simulink subsystem "Robot_Control_sub"  (R2023b)
settings: Solver=VariableStepAuto  StartTime=0.0  StopTime=10.0  RelTol=1e-3
libraries: Autonomous_lib x1, Disabled_lib x1, Teleop_lib x1, Test_lib x1
settings Model: Creator=USER  LastModifiedBy=ander

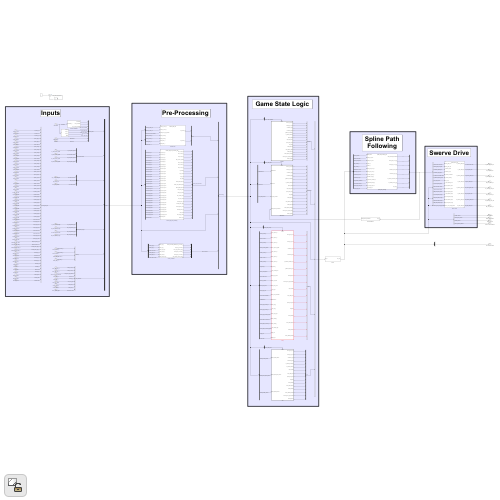
[thumbnail: Simulink's stored preview of the top-level diagram]
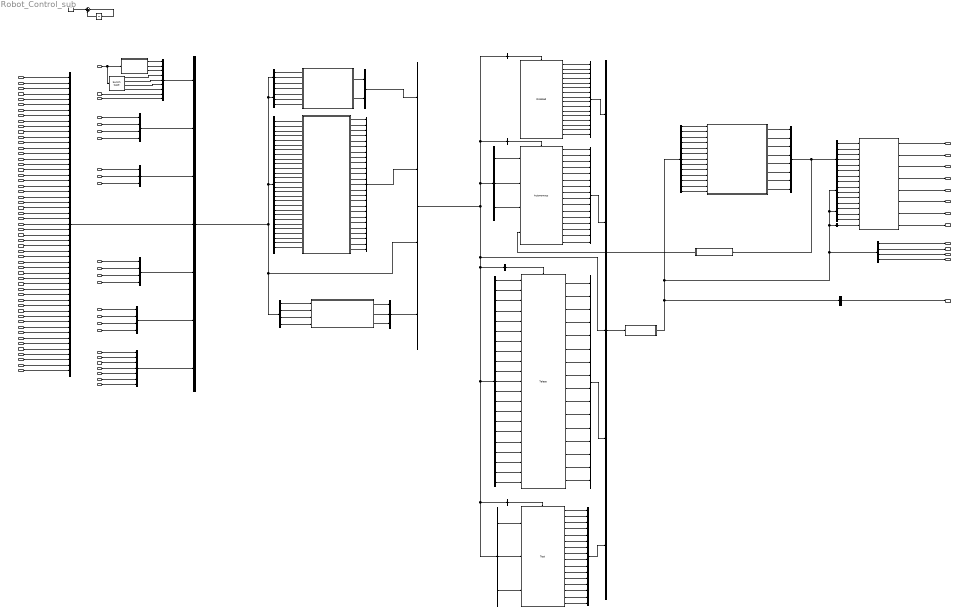
== system Robot_Control_sub ==
  note: Game State Logic
  note: Swerve Drive
  note: Inputs
  note: Pre-Processing
  note: Spline Path
      | Following
  GameState : Inport
  IsBlueAlliance : Inport  Port=2
  MatchTime : Inport  Port=3
  Joystick_Left_X : Inport  Port=4
  Joystick_Left_Y : Inport  Port=5
  Joystick_Left_Z : Inport  Port=6
  Joystick_Right_X : Inport  Port=7
  Joystick_Right_Y : Inport  Port=8
  Joystick_Right_Z : Inport  Port=9
  Joystick_Left_B1 : Inport  Port=10
  Joystick_Left_B2 : Inport  Port=11
  Joystick_Left_B3 : Inport  Port=12
  Joystick_Left_B4 : Inport  Port=13
  Joystick_Left_B5 : Inport  Port=14
  Joystick_Left_B6 : Inport  Port=15
  Joystick_Left_B7 : Inport  Port=16
  Joystick_Left_B8 : Inport  Port=17
  Joystick_Left_B9 : Inport  Port=18
  Joystick_Left_B10 : Inport  Port=19
  Joystick_Left_B11 : Inport  Port=20
  Joystick_Left_B12 : Inport  Port=21
  Joystick_Left_B13 : Inport  Port=22
  Joystick_Left_B14 : Inport  Port=23
  Joystick_Left_B15 : Inport  Port=24
  Joystick_Left_B16 : Inport  Port=25
  Joystick_Left_POV : Inport  Port=26
  Joystick_Right_B1 : Inport  Port=27
  Joystick_Right_B2 : Inport  Port=28
  Joystick_Right_B3 : Inport  Port=29
  Joystick_Right_B4 : Inport  Port=30
  Joystick_Right_B5 : Inport  Port=31
  Joystick_Right_B6 : Inport  Port=32
  Joystick_Right_B7 : Inport  Port=33
  Joystick_Right_B8 : Inport  Port=34
  Joystick_Right_B9 : Inport  Port=35
  Joystick_Right_B10 : Inport  Port=36
  Joystick_Right_B11 : Inport  Port=37
  Joystick_Right_B12 : Inport  Port=38
  Joystick_Right_B13 : Inport  Port=39
  Joystick_Right_B14 : Inport  Port=40
  Joystick_Right_B15 : Inport  Port=41
  Joystick_Right_B16 : Inport  Port=42
  Joystick_Right_POV : Inport  Port=43
  Gamepad_Stick_Left_X : Inport  Port=44
  Gamepad_Stick_Left_Y : Inport  Port=45
  Gamepad_Stick_Right_X : Inport  Port=46
  Gamepad_Stick_Right_Y : Inport  Port=47
  Gamepad_B1_A : Inport  Port=48
  Gamepad_B2_B : Inport  Port=49
  Gamepad_B3_X : Inport  Port=50
  Gamepad_B4_Y : Inport  Port=51
  Gamepad_LB : Inport  Port=52
  Gamepad_LT : Inport  Port=53
  Gamepad_RB : Inport  Port=54
  Gamepad_RT : Inport  Port=55
  Gamepad_Back : Inport  Port=56
  Gamepad_Start : Inport  Port=57
  Gamepad_POV : Inport  Port=58
  FL_Drive_Motor_Speed : Inport  Port=59
  FR_Drive_Motor_Speed : Inport  Port=60
  BL_Drive_Motor_Speed : Inport  Port=61
  BR_Drive_Motor_Speed : Inport  Port=62
  Gyro_Angle_Field_rad : Inport  Port=63
  Gyro_Angle_rad : Inport  Port=64
  Auto_Start_Position : Inport  Port=65
  FL_Steer_Module_Angle : Inport  Port=66
  FR_Steer_Module_Angle : Inport  Port=67
  BL_Steer_Module_Angle : Inport  Port=68
  BR_Steer_Module_Angle : Inport  Port=69
  Odom_Position_X : Inport  Port=70
  Odom_Position_Y : Inport  Port=71
  Odom_Delta_X : Inport  Port=72
  Odom_Delta_Y : Inport  Port=73
  Vision_Current_Pipeline : Inport  Port=74
  Vision_RobotPoseFieldSpace_X : Inport  Port=75
  Vision_RobotPoseFieldSpace_Y : Inport  Port=76
  Vision_Num_Tags_Detected : Inport  Port=77
  Vision_c1TargetPoseRobotSpace_X : Inport  Port=78
  Vision_c1TargetPoseRobotSpace_Y : Inport  Port=79
  Vision_c1TargetPoseRobotSpace_A : Inport  Port=80
  Autonomous : Autonomous_lib/Autonomous  SystemSampleTime=-1  VariantActivationTime=update diagram  AllowFlexibleInterface=on  Latency=0  AutoFrameSizeCalculation=off
  Bus Creator : BusCreator  Inputs=9
  Bus Creator{1..2,4,12} (4 alike) : BusCreator  Inputs=16
  Bus Creator11 : BusCreator  Inputs=7
  Bus Creator13 : BusCreator  Inputs=8
  Bus Creator14 : BusCreator  Inputs=3
  Bus Creator{7..9,17} (4 alike) : BusCreator  Inputs=4
  Bus Creator18 : BusCreator  Inputs=7
  Bus Creator19 : BusCreator  Inputs=2
  Bus Creator21 : BusCreator  Inputs=3
  Bus Creator24 : BusCreator  Inputs=25
  Bus Creator3 : BusCreator  Inputs=5
  Bus Creator5 : BusCreator  Inputs=55
  Bus Selector : BusSelector  OutputSignals=Steering_Abs_Cmd_SPF,Steering_Rel_Cmd_SPF,Translation_Speed_SPF,Translation_Angle_SPF,Is_Absolute_Translation_SPF,Is_Absolute_Steering_SPF,Gyro_Angle_SPF
  Bus Selector1 : BusSelector  OutputSignals=Odometry.Odom_Position_X,Odometry.Odom_Position_Y,Odometry.Odom_Delta_X,Odometry.Odom_Delta_Y
  Bus Selector13 : BusSelector  OutputSignals=Human_Inputs_Raw.Joystick_Left_X,Human_Inputs_Raw.Joystick_Left_Y,Human_Inputs_Raw.Joystick_Left_Z,Human_Inputs_Raw.Joystick_Right_X,Human_Inputs_Raw.Joystick_Right_Y,Human_Inputs_Raw.Joystick_Right_Z,Human_Inputs_Raw.Joystick_Left_B1,Human_Inputs_Raw.Joystick_Left_B2,Human_Inputs_Raw.Joystick_Left_B3,Human_Inputs_Raw.Joystick_Left_B4,Human_Inputs_Raw.Joystick_Left_B5,Human_Inputs_Raw.Joystick_Left_B7,Human_Inputs_Raw.Joystick_Left_B8,Human_Inputs_Raw.Joystick_Left_B11,Human_Inputs_Raw.Joystick_Left_B12,Human_Inputs_Raw.Joystick_Left_B13,Human_Inputs_Raw.Joystick_Left_POV,Human_Inputs_Raw.Joystick_Right_B2,Human_Inputs_Raw.Joystick_Right_B3,Human_Inputs_Raw.Joystick_Right_B4,Human_Inputs_Raw.Joystick_Right_B5,Human_Inputs_Raw.Joystick_Right_B6,Human_Inputs_Raw.Joystick_Right_B7,Human_Inputs_Raw.Joystick_Right_B8,Human_Inputs_Raw.Joystick_Right_B9,Human_Inputs_Raw.Joystick_Right_B10,Human_Inputs_Raw.Joystick_Right_POV,Human_Inputs_Raw.Gamepad_POV
  Bus Selector16 : BusSelector  OutputSignals=Human_Inputs_Processed.Button_Enable_Wheels,Human_Inputs_Processed.Button_Reset_Wheel_Offsets,Human_Inputs_Processed.Button_Disable_Wheels
  Bus Selector18 : BusSelector  OutputSignals=Enable_Wheels,Reset_Wheel_Offsets,Disable_Wheels,Swerve_Motors_Disabled
  Bus Selector2 : BusSelector  OutputSignals=Inputs.Game_States.Game_State_Teleop
  Bus Selector20 : BusSelector  OutputSignals=Vision_Estimates.Vision_Current_Pipeline,Vision_Estimates.Vision_c1TargetPoseRobotSpace_X,Vision_Estimates.Vision_c1TargetPoseRobotSpace_Y,Vision_Estimates.Vision_c1TargetPoseRobotSpace_A
  Bus Selector21 : BusSelector  OutputSignals=Swerve_Drive_Integral_Enable
  Bus Selector23 : BusSelector  OutputSignals=Desired_Pipeline  OutputAsBus=on
  Bus Selector3 : BusSelector  OutputSignals=Vision_Estimates.Vision_RobotPoseFieldSpace_X,Vision_Estimates.Vision_RobotPoseFieldSpace_Y,Vision_Estimates.Vision_Num_Tags_Detected
  Bus Selector4 : BusSelector  OutputSignals=Inputs.Game_States.Game_State_Auto
  Bus Selector41 : BusSelector  OutputSignals=Human_Inputs_Processed.Drive_Joystick_X,Human_Inputs_Processed.Drive_Joystick_Y,Human_Inputs_Processed.Drive_Joystick_Z,Human_Inputs_Processed.Drive_Joystick_Z_Mode,Human_Inputs_Processed.Steer_Joystick_X,Human_Inputs_Processed.Steer_Joystick_Y,Human_Inputs_Processed.Steer_Joystick_Z,Human_Inputs_Processed.Is_Boosting,Human_Inputs_Processed.Face_Toward_Driver,Human_Inputs_Processed.Face_Right_Driver,Human_Inputs_Processed.Face_Left_Driver,Human_Inputs_Processed.Face_Away_Driver,Inputs.Gyro.Gyro_Angle_rad,Inputs.Game_States.Prev_Active_GameState,Inputs.Game_States.IsBlueAlliance,Inputs.Vision_Estimates.Vision_Current_Pipeline,Vision_Corrected.Vision_c1TPRS_Corrected_X,Vision_Corrected.Vision_c1TPRS_Corrected_Y,Vision_Corrected.Vision_c1TPRS_Corrected_A,Human_Inputs_Processed.Align_Left,Human_Inputs_Processed.Align_Right
  Bus Selector50 : BusSelector  OutputSignals=PreProcessing.Inputs.Drive_Motor_Speeds.FL_Drive_Motor_Speed,PreProcessing.Inputs.Drive_Motor_Speeds.FR_Drive_Motor_Speed,PreProcessing.Inputs.Drive_Motor_Speeds.BL_Drive_Motor_Speed,PreProcessing.Inputs.Drive_Motor_Speeds.BR_Drive_Motor_Speed
  Bus Selector52 : BusSelector  OutputSignals=PreProcessing.Inputs.Steer_Module_Angles.FL_Steer_Module_Angle,PreProcessing.Inputs.Steer_Module_Angles.FR_Steer_Module_Angle,PreProcessing.Inputs.Steer_Module_Angles.BL_Steer_Module_Angle,PreProcessing.Inputs.Steer_Module_Angles.BR_Steer_Module_Angle
  Bus Selector59 : BusSelector  OutputSignals=Inputs.Game_States.IsBlueAlliance,Inputs.Game_States.MatchTime,Inputs.Gyro.Auto_Start_Position
  Bus Selector6 : BusSelector  OutputSignals=Inputs.Game_States.Game_State_Disabled
  Bus Selector8 : BusSelector  OutputSignals=Inputs.Game_States.Game_State_Test
  Bus Selector9 : BusSelector  OutputSignals=Spline_Enable,Spline_Ref_Poses,Spline_Num_Poses,PreProcessing.EKF.KF_Position_X,PreProcessing.EKF.KF_Position_Y,Steering_Abs_Cmd,Steering_Rel_Cmd,Translation_Speed,Translation_Angle,Is_Absolute_Translation,Is_Absolute_Steering,PreProcessing.Inputs.Gyro.Gyro_Angle_Field_rad,PreProcessing.Inputs.Gyro.Gyro_Angle_rad
  Constant2 : Constant
  Disabled : Disabled_lib/Disabled  SystemSampleTime=-1  VariantActivationTime=update diagram  AllowFlexibleInterface=on  Latency=0  AutoFrameSizeCalculation=off
  Human_Input_Pre_Processing : Subsystem  ReferencedSubsystem=Human_Input_Pre_Processing_sub
  Internal Feedback : Subsystem
  Kalman_Filter : Subsystem  ReferencedSubsystem=Kalman_Filter_sub
  Merge : Subsystem
  Previous GameState : Subsystem
  Spline_Path_Following : Subsystem  ReferencedSubsystem=Spline_Path_Following_sub
  Sum : Sum  Inputs=|++
  Swerve_Drive : Subsystem  ReferencedSubsystem=Swerve_Drive_sub
  Switch Case : SwitchCase  CaseConditions={0,1,2}
  Teleop : Teleop_lib/Teleop  SystemSampleTime=-1  VariantActivationTime=update diagram  AllowFlexibleInterface=on  Latency=0  AutoFrameSizeCalculation=off
  Test : Test_lib/Test  SystemSampleTime=-1  VariantActivationTime=update diagram  AllowFlexibleInterface=on  Latency=0  AutoFrameSizeCalculation=off
  Unit Delay1 : UnitDelay  SampleTime=-1  HasFrameUpgradeWarning=on
  Vision_Corrections : Subsystem  ReferencedSubsystem=Vision_Corrections_sub
  FL_Steering_Motor_DC : Outport
  FL_Drive_Motor_DC : Outport  Port=2
  FR_Steering_Motor_DC : Outport  Port=3
  FR_Drive_Motor_DC : Outport  Port=4
  BL_Steering_Motor_DC : Outport  Port=5
  BL_Drive_Motor_DC : Outport  Port=6
  BR_Steering_Motor_DC : Outport  Port=7
  BR_Drive_Motor_DC : Outport  Port=8
  Enable_Wheels : Outport  Port=9
  Reset_Wheel_Offsets : Outport  Port=10
  Disable_Wheels : Outport  Port=11
  Swerve_Motors_Disabled : Outport  Port=12
  Vision_Desired_Pipeline : Outport  Port=13
  wires:
  Bus Creator4/1 -> Bus Creator3/1  "Disabled"
  Bus Creator1/1 -> Bus Creator3/2  "Autonomous"
  Bus Creator2/1 -> Bus Creator3/4  "Teleop"
  Switch Case/1 -> Bus Creator/4  "Game_State_Disabled"
  Switch Case/2 -> Bus Creator/5  "Game_State_Auto"
  Switch Case/3 -> Bus Creator/6  "Game_State_Teleop"
  GameState/1 -> Previous GameState/1(GameState_in), Switch Case/1  "GameState"
  Bus Creator12/1 -> Bus Creator3/5  "Test"
  Switch Case/4 -> Bus Creator/7  "Game_State_Test"
  FL_Drive_Motor_Speed/1 -> Bus Creator7/1  "FL_Drive_Motor_Speed"
  FR_Drive_Motor_Speed/1 -> Bus Creator7/2  "FR_Drive_Motor_Speed"
  BL_Drive_Motor_Speed/1 -> Bus Creator7/3  "BL_Drive_Motor_Speed"
  BR_Drive_Motor_Speed/1 -> Bus Creator7/4  "BR_Drive_Motor_Speed"
  Bus Creator/1 -> Bus Creator11/1  "Game_States"
  Bus Selector2/1 -> Teleop/Action  "<Game_State_Teleop>"
  Bus Selector4/1 -> Autonomous/Action  "<Game_State_Auto>"
  Bus Selector6/1 -> Disabled/Action  "<Game_State_Disabled>"
  Bus Selector8/1 -> Test/Action  "<Game_State_Test>"
  Bus Selector50/4 -> Swerve_Drive/11  "<BR_Drive_Motor_Speed>"
  Bus Selector50/3 -> Swerve_Drive/10  "<BL_Drive_Motor_Speed>"
  Bus Selector50/2 -> Swerve_Drive/9  "<FR_Drive_Motor_Speed>"
  Bus Selector50/1 -> Swerve_Drive/8  "<FL_Drive_Motor_Speed>"
  Swerve_Drive/1 -> FL_Steering_Motor_DC/1
  Swerve_Drive/2 -> FL_Drive_Motor_DC/1
  Swerve_Drive/3 -> FR_Steering_Motor_DC/1
  Swerve_Drive/4 -> FR_Drive_Motor_DC/1
  Swerve_Drive/5 -> BL_Steering_Motor_DC/1
  Swerve_Drive/6 -> BL_Drive_Motor_DC/1
  Swerve_Drive/7 -> BR_Steering_Motor_DC/1
  Swerve_Drive/8 -> BR_Drive_Motor_DC/1
  Joystick_Left_B1/1 -> Bus Creator5/7  "Joystick_Left_B1"
  Gyro_Angle_Field_rad/1 -> Bus Creator14/1  "Gyro_Angle_Field_rad"
  Gyro_Angle_rad/1 -> Bus Creator14/2  "Gyro_Angle_rad"
  Bus Creator11/1 -> Bus Creator17/3, Bus Selector20/1, Bus Selector1/1, Bus Selector3/1, Bus Selector13/1  "Inputs"
  Bus Selector52/1 -> Swerve_Drive/12  "<FL_Steer_Module_Angle>"
  Bus Selector52/2 -> Swerve_Drive/13  "<FR_Steer_Module_Angle>"
  Bus Selector52/3 -> Swerve_Drive/14  "<BL_Steer_Module_Angle>"
  Bus Selector52/4 -> Swerve_Drive/15  "<BR_Steer_Module_Angle>"
  Merge/1(Bus_Out) -> Bus Selector23/1, Bus Selector9/1, Bus Selector18/1, Bus Selector21/1, Bus Selector52/1, Bus Selector50/1
  Bus Creator3/1 -> Merge/1(Bus_In)
  Bus Selector9/1 -> Spline_Path_Following/1  "<Spline_Enable>"
  Bus Selector9/2 -> Spline_Path_Following/2  "<Spline_Ref_Poses>"
  Bus Selector9/3 -> Spline_Path_Following/3  "<Spline_Num_Poses>"
  Bus Selector9/6 -> Spline_Path_Following/6  "<Steering_Abs_Cmd>"
  Bus Selector9/7 -> Spline_Path_Following/7  "<Steering_Rel_Cmd>"
  Bus Selector9/8 -> Spline_Path_Following/8  "<Translation_Speed>"
  Bus Selector9/9 -> Spline_Path_Following/9  "<Translation_Angle>"
  Bus Selector9/10 -> Spline_Path_Following/10  "<Is_Absolute_Translation>"
  Bus Selector9/11 -> Spline_Path_Following/11  "<Is_Absolute_Steering>"
  Spline_Path_Following/2 -> Bus Creator13/2
  Spline_Path_Following/3 -> Bus Creator13/3
  Spline_Path_Following/4 -> Bus Creator13/4
  Spline_Path_Following/5 -> Bus Creator13/5
  Spline_Path_Following/6 -> Bus Creator13/6
  Spline_Path_Following/7 -> Bus Creator13/7
  Bus Creator13/1 -> Bus Selector/1, Internal Feedback/1(Bus_In)
  Bus Selector/5 -> Swerve_Drive/5  "<Is_Absolute_Translation_SPF>"
  Bus Selector/4 -> Swerve_Drive/4  "<Translation_Angle_SPF>"
  Bus Selector/6 -> Swerve_Drive/6  "<Is_Absolute_Steering_SPF>"
  Bus Selector/3 -> Swerve_Drive/3  "<Translation_Speed_SPF>"
  Bus Selector/2 -> Swerve_Drive/2  "<Steering_Rel_Cmd_SPF>"
  Bus Selector/1 -> Swerve_Drive/1  "<Steering_Abs_Cmd_SPF>"
  Spline_Path_Following/1 -> Bus Creator13/1
  Vision_RobotPoseFieldSpace_X/1 -> Bus Creator18/2  "Vision_RobotPoseFieldSpace_X"
  Vision_RobotPoseFieldSpace_Y/1 -> Bus Creator18/3  "Vision_RobotPoseFieldSpace_Y"
  Vision_Num_Tags_Detected/1 -> Bus Creator18/4  "Vision_Num_Tags_Detected"
  Bus Selector1/3 -> Kalman_Filter/6  "<Odom_Delta_X>"
  Bus Selector1/4 -> Kalman_Filter/7  "<Odom_Delta_Y>"
  Bus Selector3/3 -> Kalman_Filter/3  "<Vision_Num_Tags_Detected>"
  Bus Selector3/2 -> Kalman_Filter/2  "<Vision_RobotPoseFieldSpace_Y>"
  Bus Selector3/1 -> Kalman_Filter/1  "<Vision_RobotPoseFieldSpace_X>"
  Kalman_Filter/1 -> Bus Creator19/1
  Kalman_Filter/2 -> Bus Creator19/2
  Bus Selector9/4 -> Spline_Path_Following/4  "<KF_Position_X>"
  Bus Selector9/5 -> Spline_Path_Following/5  "<KF_Position_Y>"
  Bus Creator19/1 -> Bus Creator17/1  "EKF"
  Bus Selector1/2 -> Kalman_Filter/5  "<Odom_Position_Y>"
  Bus Selector1/1 -> Kalman_Filter/4  "<Odom_Position_X>"
  Joystick_Left_B4/1 -> Bus Creator5/10  "Joystick_Left_B4"
  Joystick_Left_B3/1 -> Bus Creator5/9  "Joystick_Left_B3"
  Joystick_Left_B2/1 -> Bus Creator5/8  "Joystick_Left_B2"
  Bus Selector13/4 -> Human_Input_Pre_Processing/4  "<Joystick_Right_X>"
  Bus Selector13/5 -> Human_Input_Pre_Processing/5  "<Joystick_Right_Y>"
  Bus Selector13/1 -> Human_Input_Pre_Processing/1  "<Joystick_Left_X>"
  Bus Selector13/3 -> Human_Input_Pre_Processing/3  "<Joystick_Left_Z>"
  Bus Selector13/2 -> Human_Input_Pre_Processing/2  "<Joystick_Left_Y>"
  Bus Selector13/6 -> Human_Input_Pre_Processing/6  "<Joystick_Right_Z>"
  Bus Selector13/7 -> Human_Input_Pre_Processing/7  "<Joystick_Left_B1>"
  Bus Selector13/8 -> Human_Input_Pre_Processing/8  "<Joystick_Left_B2>"
  Bus Selector13/9 -> Human_Input_Pre_Processing/9  "<Joystick_Left_B3>"
  Bus Selector13/10 -> Human_Input_Pre_Processing/10  "<Joystick_Left_B4>"
  Joystick_Left_Y/1 -> Bus Creator5/2  "Joystick_Left_Y"
  Joystick_Left_X/1 -> Bus Creator5/1  "Joystick_Left_X"
  Joystick_Left_Z/1 -> Bus Creator5/3  "Joystick_Left_Z"
  Joystick_Right_X/1 -> Bus Creator5/4  "Joystick_Right_X"
  Joystick_Right_Y/1 -> Bus Creator5/5  "Joystick_Right_Y"
  Joystick_Right_Z/1 -> Bus Creator5/6  "Joystick_Right_Z"
  Bus Creator24/1 -> Bus Creator17/2  "Human_Inputs_Processed"
  Bus Creator17/1 -> Bus Selector59/1, Bus Selector4/1, Bus Selector6/1, Bus Creator3/3, Bus Selector2/1, Bus Selector41/1, Bus Selector8/1, Bus Selector16/1  "PreProcessing"
  Bus Creator18/1 -> Bus Creator11/7  "Vision_Estimates"
  Internal Feedback/1(Robot_Reached_Destination) -> Autonomous/4
  Vision_c1TargetPoseRobotSpace_X/1 -> Bus Creator18/5  "Vision_c1TargetPoseRobotSpace_X"
  Vision_c1TargetPoseRobotSpace_Y/1 -> Bus Creator18/6  "Vision_c1TargetPoseRobotSpace_Y"
  Previous GameState/1(GameState) -> Bus Creator/1
  Previous GameState/3(Prev_Active_GameState) -> Bus Creator/3
  IsBlueAlliance/1 -> Bus Creator/8  "IsBlueAlliance"
  Bus Selector9/12 -> Spline_Path_Following/12  "<Gyro_Angle_Field_rad>"
  Bus Selector9/13 -> Spline_Path_Following/13  "<Gyro_Angle_rad>"
  Spline_Path_Following/8 -> Bus Creator13/8
  Bus Selector/7 -> Swerve_Drive/7  "<Gyro_Angle_SPF>"
  Bus Selector59/1 -> Autonomous/1  "<IsBlueAlliance>"
  Bus Selector18/2 -> Reset_Wheel_Offsets/1  "<Reset_Wheel_Offsets>"
  Bus Selector18/3 -> Disable_Wheels/1  "<Disable_Wheels>"
  Bus Selector18/4 -> Swerve_Motors_Disabled/1  "<Swerve_Motors_Disabled>"
  Bus Selector18/1 -> Enable_Wheels/1  "<Enable_Wheels>"
  Bus Selector16/1 -> Test/1  "<Button_Enable_Wheels>"
  Bus Selector16/2 -> Test/2  "<Button_Reset_Wheel_Offsets>"
  Bus Selector16/3 -> Test/3  "<Button_Disable_Wheels>"
  Joystick_Left_B5/1 -> Bus Creator5/11  "Joystick_Left_B5"
  Joystick_Left_B6/1 -> Bus Creator5/12  "Joystick_Left_B6"
  Joystick_Left_B7/1 -> Bus Creator5/13  "Joystick_Left_B7"
  Joystick_Left_B8/1 -> Bus Creator5/14  "Joystick_Left_B8"
  Joystick_Left_B9/1 -> Bus Creator5/15  "Joystick_Left_B9"
  Joystick_Left_B10/1 -> Bus Creator5/16  "Joystick_Left_B10"
  Joystick_Left_B11/1 -> Bus Creator5/17  "Joystick_Left_B11"
  Joystick_Left_B12/1 -> Bus Creator5/18  "Joystick_Left_B12"
  Joystick_Left_B13/1 -> Bus Creator5/19  "Joystick_Left_B13"
  Joystick_Left_B14/1 -> Bus Creator5/20  "Joystick_Left_B14"
  Joystick_Left_B15/1 -> Bus Creator5/21  "Joystick_Left_B15"
  Joystick_Left_B16/1 -> Bus Creator5/22  "Joystick_Left_B16"
  Joystick_Left_POV/1 -> Bus Creator5/23  "Joystick_Left_POV"
  Joystick_Right_B1/1 -> Bus Creator5/24  "Joystick_Right_B1"
  Joystick_Right_B2/1 -> Bus Creator5/25  "Joystick_Right_B2"
  Joystick_Right_B3/1 -> Bus Creator5/26  "Joystick_Right_B3"
  Joystick_Right_B4/1 -> Bus Creator5/27  "Joystick_Right_B4"
  Joystick_Right_B5/1 -> Bus Creator5/28  "Joystick_Right_B5"
  Joystick_Right_B6/1 -> Bus Creator5/29  "Joystick_Right_B6"
  Joystick_Right_B7/1 -> Bus Creator5/30  "Joystick_Right_B7"
  Joystick_Right_B8/1 -> Bus Creator5/31  "Joystick_Right_B8"
  Joystick_Right_B9/1 -> Bus Creator5/32  "Joystick_Right_B9"
  Joystick_Right_B10/1 -> Bus Creator5/33  "Joystick_Right_B10"
  Joystick_Right_B11/1 -> Bus Creator5/34  "Joystick_Right_B11"
  Joystick_Right_B12/1 -> Bus Creator5/35  "Joystick_Right_B12"
  Joystick_Right_B13/1 -> Bus Creator5/36  "Joystick_Right_B13"
  Joystick_Right_B14/1 -> Bus Creator5/37  "Joystick_Right_B14"
  Joystick_Right_B15/1 -> Bus Creator5/38  "Joystick_Right_B15"
  Joystick_Right_B16/1 -> Bus Creator5/39  "Joystick_Right_B16"
  Joystick_Right_POV/1 -> Bus Creator5/40  "Joystick_Right_POV"
  Gamepad_Stick_Left_X/1 -> Bus Creator5/41  "Gamepad_Stick_Left_X"
  Gamepad_Stick_Left_Y/1 -> Bus Creator5/42  "Gamepad_Stick_Left_Y"
  Gamepad_Stick_Right_X/1 -> Bus Creator5/43  "Gamepad_Stick_Right_X"
  Gamepad_Stick_Right_Y/1 -> Bus Creator5/44  "Gamepad_Stick_Right_Y"
  Gamepad_B1_A/1 -> Bus Creator5/45  "Gamepad_B1_A"
  Gamepad_B2_B/1 -> Bus Creator5/46  "Gamepad_B2_B"
  Gamepad_B3_X/1 -> Bus Creator5/47  "Gamepad_B3_X"
  Gamepad_B4_Y/1 -> Bus Creator5/48  "Gamepad_B4_Y"
  Gamepad_LB/1 -> Bus Creator5/49  "Gamepad_LB"
  Gamepad_LT/1 -> Bus Creator5/50  "Gamepad_LT"
  Gamepad_RB/1 -> Bus Creator5/51  "Gamepad_RB"
  Gamepad_RT/1 -> Bus Creator5/52  "Gamepad_RT"
  Gamepad_Back/1 -> Bus Creator5/53  "Gamepad_Back"
  Gamepad_Start/1 -> Bus Creator5/54  "Gamepad_Start"
  Bus Creator5/1 -> Bus Creator11/4  "Human_Inputs_Raw"
  Gamepad_POV/1 -> Bus Creator5/55  "Gamepad_POV"
  Vision_Corrections/1 -> Bus Creator21/1
  Vision_Corrections/2 -> Bus Creator21/2
  Vision_Corrections/3 -> Bus Creator21/3
  Bus Creator21/1 -> Bus Creator17/4  "Vision_Corrected"
  Human_Input_Pre_Processing/1 -> Bus Creator24/1
  Human_Input_Pre_Processing/2 -> Bus Creator24/2
  Human_Input_Pre_Processing/3 -> Bus Creator24/3
  Human_Input_Pre_Processing/4 -> Bus Creator24/4
  Human_Input_Pre_Processing/5 -> Bus Creator24/5
  Human_Input_Pre_Processing/6 -> Bus Creator24/6
  Human_Input_Pre_Processing/7 -> Bus Creator24/7
  Human_Input_Pre_Processing/8 -> Bus Creator24/8
  Human_Input_Pre_Processing/9 -> Bus Creator24/9
  Human_Input_Pre_Processing/10 -> Bus Creator24/10
  Human_Input_Pre_Processing/11 -> Bus Creator24/11
  Bus Selector41/1 -> Teleop/1  "<Drive_Joystick_X>"
  Bus Selector13/14 -> Human_Input_Pre_Processing/14  "<Joystick_Left_B11>"
  Bus Selector13/15 -> Human_Input_Pre_Processing/15  "<Joystick_Left_B12>"
  Bus Selector13/16 -> Human_Input_Pre_Processing/16  "<Joystick_Left_B13>"
  Bus Selector13/17 -> Human_Input_Pre_Processing/17  "<Joystick_Left_POV>"
  Bus Selector13/18 -> Human_Input_Pre_Processing/18  "<Joystick_Right_B2>"
  Bus Selector13/19 -> Human_Input_Pre_Processing/19  "<Joystick_Right_B3>"
  Bus Selector13/20 -> Human_Input_Pre_Processing/20  "<Joystick_Right_B4>"
  Bus Selector13/21 -> Human_Input_Pre_Processing/21  "<Joystick_Right_B5>"
  Bus Selector13/22 -> Human_Input_Pre_Processing/22  "<Joystick_Right_B6>"
  Bus Selector13/23 -> Human_Input_Pre_Processing/23  "<Joystick_Right_B7>"
  Bus Selector13/24 -> Human_Input_Pre_Processing/24  "<Joystick_Right_B8>"
  Bus Selector13/25 -> Human_Input_Pre_Processing/25  "<Joystick_Right_B9>"
  Bus Selector13/26 -> Human_Input_Pre_Processing/26  "<Joystick_Right_B10>"
  Bus Selector13/27 -> Human_Input_Pre_Processing/27  "<Joystick_Right_POV>"
  Bus Selector13/28 -> Human_Input_Pre_Processing/28  "<Gamepad_POV>"
  Bus Selector41/2 -> Teleop/2  "<Drive_Joystick_Y>"
  Bus Selector41/3 -> Teleop/3  "<Drive_Joystick_Z>"
  Bus Selector41/4 -> Teleop/4  "<Drive_Joystick_Z_Mode>"
  Bus Selector41/5 -> Teleop/5  "<Steer_Joystick_X>"
  Bus Selector41/6 -> Teleop/6  "<Steer_Joystick_Y>"
  Bus Selector41/7 -> Teleop/7  "<Steer_Joystick_Z>"
  Bus Selector41/8 -> Teleop/8  "<Is_Boosting>"
  Bus Selector41/9 -> Teleop/9  "<Face_Toward_Driver>"
  Bus Selector41/10 -> Teleop/10  "<Face_Right_Driver>"
  Bus Selector41/11 -> Teleop/11  "<Face_Left_Driver>"
  Bus Selector41/12 -> Teleop/12  "<Face_Away_Driver>"
  Bus Selector41/13 -> Teleop/13  "<Gyro_Angle_rad>"
  Bus Selector21/1 -> Swerve_Drive/16  "<Swerve_Drive_Integral_Enable>"
  Previous GameState/2(Prev_GameState) -> Bus Creator/2
  Bus Selector41/14 -> Teleop/14  "<Prev_Active_GameState>"
  Bus Selector41/15 -> Teleop/15  "<IsBlueAlliance>"
  Bus Selector13/11 -> Human_Input_Pre_Processing/11  "<Joystick_Left_B5>"
  Bus Selector13/12 -> Human_Input_Pre_Processing/12  "<Joystick_Left_B7>"
  Bus Selector13/13 -> Human_Input_Pre_Processing/13  "<Joystick_Left_B8>"
  MatchTime/1 -> Bus Creator/9  "MatchTime"
  Bus Selector41/17 -> Teleop/17  "<Vision_c1TPRS_Corrected_X>"
  Bus Selector41/18 -> Teleop/18  "<Vision_c1TPRS_Corrected_Y>"
  Bus Selector41/19 -> Teleop/19  "<Vision_c1TPRS_Corrected_A>"
  Human_Input_Pre_Processing/12 -> Bus Creator24/12
  Human_Input_Pre_Processing/13 -> Bus Creator24/13
  Human_Input_Pre_Processing/14 -> Bus Creator24/14
  Human_Input_Pre_Processing/15 -> Bus Creator24/15
  Human_Input_Pre_Processing/16 -> Bus Creator24/16
  Human_Input_Pre_Processing/17 -> Bus Creator24/17
  Human_Input_Pre_Processing/18 -> Bus Creator24/18
  Human_Input_Pre_Processing/19 -> Bus Creator24/19
  Human_Input_Pre_Processing/20 -> Bus Creator24/20
  Human_Input_Pre_Processing/21 -> Bus Creator24/21
  Human_Input_Pre_Processing/22 -> Bus Creator24/22
  Human_Input_Pre_Processing/23 -> Bus Creator24/23
  Human_Input_Pre_Processing/24 -> Bus Creator24/24
  Human_Input_Pre_Processing/25 -> Bus Creator24/25
  Bus Selector59/2 -> Autonomous/2  "<MatchTime>"
  Bus Selector23/1 -> Vision_Desired_Pipeline/1
  Odom_Position_X/1 -> Bus Creator9/1  "Odom_Position_X"
  Odom_Position_Y/1 -> Bus Creator9/2  "Odom_Position_Y"
  Odom_Delta_X/1 -> Bus Creator9/3  "Odom_Delta_X"
  Odom_Delta_Y/1 -> Bus Creator9/4  "Odom_Delta_Y"
  Bus Creator9/1 -> Bus Creator11/6  "Odometry"
  BR_Steer_Module_Angle/1 -> Bus Creator8/4  "BR_Steer_Module_Angle"
  BL_Steer_Module_Angle/1 -> Bus Creator8/3  "BL_Steer_Module_Angle"
  FR_Steer_Module_Angle/1 -> Bus Creator8/2  "FR_Steer_Module_Angle"
  FL_Steer_Module_Angle/1 -> Bus Creator8/1  "FL_Steer_Module_Angle"
  Bus Creator7/1 -> Bus Creator11/2  "Drive_Motor_Speeds"
  Bus Creator14/1 -> Bus Creator11/3  "Gyro"
  Auto_Start_Position/1 -> Bus Creator14/3  "Auto_Start_Position"
  Constant2/1 -> Sum/1
  Unit Delay1/1 -> Sum/2
  Sum/1 -> Unit Delay1/1  "loop_counter_robot_control"
  Vision_c1TargetPoseRobotSpace_A/1 -> Bus Creator18/7  "Vision_c1TargetPoseRobotSpace_A"
  Teleop/1 -> Bus Creator2/1
  Teleop/2 -> Bus Creator2/2
  Teleop/3 -> Bus Creator2/3
  Teleop/4 -> Bus Creator2/4
  Teleop/5 -> Bus Creator2/5
  Teleop/6 -> Bus Creator2/6
  Teleop/7 -> Bus Creator2/7
  Teleop/8 -> Bus Creator2/8
  Teleop/9 -> Bus Creator2/9
  Teleop/10 -> Bus Creator2/10
  Teleop/11 -> Bus Creator2/11
  Teleop/12 -> Bus Creator2/12
  Teleop/13 -> Bus Creator2/13
  Teleop/14 -> Bus Creator2/14
  Teleop/15 -> Bus Creator2/15
  Teleop/16 -> Bus Creator2/16
  Bus Selector41/20 -> Teleop/20  "<Align_Left>"
  Bus Selector41/21 -> Teleop/21  "<Align_Right>"
  Test/1 -> Bus Creator12/1
  Test/2 -> Bus Creator12/2
  Test/3 -> Bus Creator12/3
  Test/4 -> Bus Creator12/4
  Test/5 -> Bus Creator12/5
  Test/6 -> Bus Creator12/6
  Test/7 -> Bus Creator12/7
  Test/8 -> Bus Creator12/8
  Test/9 -> Bus Creator12/9
  Test/10 -> Bus Creator12/10
  Test/11 -> Bus Creator12/11
  Test/12 -> Bus Creator12/12
  Test/13 -> Bus Creator12/13
  Test/14 -> Bus Creator12/14
  Test/15 -> Bus Creator12/15
  Test/16 -> Bus Creator12/16
  Disabled/1 -> Bus Creator4/1
  Disabled/2 -> Bus Creator4/2
  Disabled/3 -> Bus Creator4/3
  Disabled/4 -> Bus Creator4/4
  Disabled/5 -> Bus Creator4/5
  Disabled/6 -> Bus Creator4/6
  Disabled/7 -> Bus Creator4/7
  Disabled/8 -> Bus Creator4/8
  Disabled/9 -> Bus Creator4/9
  Disabled/10 -> Bus Creator4/10
  Disabled/11 -> Bus Creator4/11
  Disabled/12 -> Bus Creator4/12
  Disabled/13 -> Bus Creator4/13
  Disabled/14 -> Bus Creator4/14
  Disabled/15 -> Bus Creator4/15
  Disabled/16 -> Bus Creator4/16
  Bus Selector59/3 -> Autonomous/3  "<Auto_Start_Position>"
  Autonomous/1 -> Bus Creator1/1
  Autonomous/2 -> Bus Creator1/2
  Autonomous/3 -> Bus Creator1/3
  Autonomous/4 -> Bus Creator1/4
  Autonomous/5 -> Bus Creator1/5
  Autonomous/6 -> Bus Creator1/6
  Autonomous/7 -> Bus Creator1/7
  Autonomous/8 -> Bus Creator1/8
  Autonomous/9 -> Bus Creator1/9
  Autonomous/10 -> Bus Creator1/10
  Autonomous/11 -> Bus Creator1/11
  Autonomous/12 -> Bus Creator1/12
  Autonomous/13 -> Bus Creator1/13
  Autonomous/14 -> Bus Creator1/14
  Autonomous/15 -> Bus Creator1/15
  Autonomous/16 -> Bus Creator1/16
  Bus Creator8/1 -> Bus Creator11/5  "Steer_Module_Angles"
  Vision_Current_Pipeline/1 -> Bus Creator18/1  "Vision_Current_Pipeline"
  Bus Selector20/2 -> Vision_Corrections/2  "<Vision_c1TargetPoseRobotSpace_X>"
  Bus Selector20/3 -> Vision_Corrections/3  "<Vision_c1TargetPoseRobotSpace_Y>"
  Bus Selector20/4 -> Vision_Corrections/4  "<Vision_c1TargetPoseRobotSpace_A>"
  Bus Selector20/1 -> Vision_Corrections/1  "<Vision_Current_Pipeline>"
  Bus Selector41/16 -> Teleop/16  "<Vision_Current_Pipeline>"

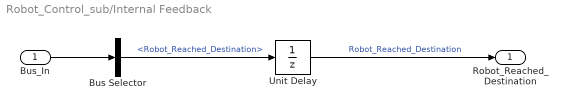
== system Robot_Control_sub/Internal Feedback ==
  Bus_In : Inport
  Bus Selector : BusSelector  OutputSignals=Robot_Reached_Destination
  Unit Delay : UnitDelay  SampleTime=-1  HasFrameUpgradeWarning=on
  Robot_Reached_Destination : Outport
  wires:
  Unit Delay/1 -> Robot_Reached_Destination/1  "Robot_Reached_Destination"
  Bus Selector/1 -> Unit Delay/1  "<Robot_Reached_Destination>"
  Bus_In/1 -> Bus Selector/1

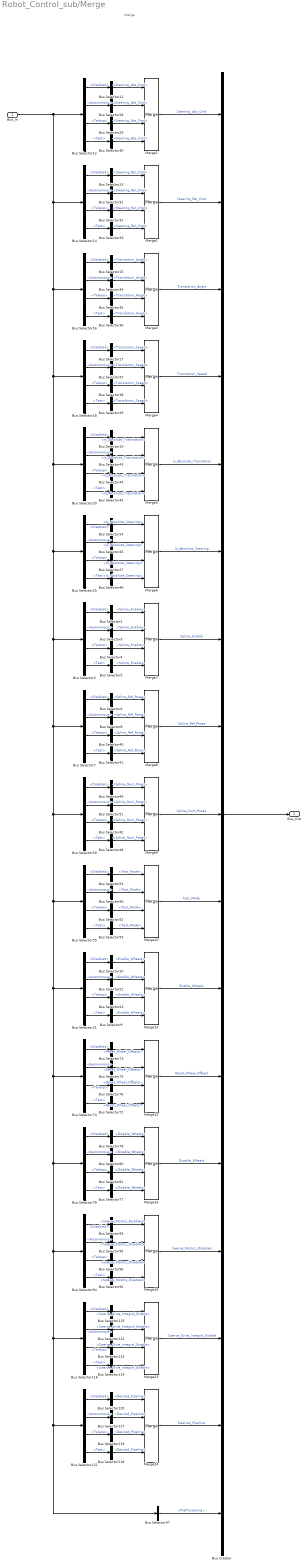
== system Robot_Control_sub/Merge ==
  note: Merge
  Bus_In : Inport
  Bus Creator : BusCreator  Inputs=17
  Bus Selector{1,3..5} (4 alike) : BusSelector  OutputSignals=Spline_Enable
  Bus Selector{9..10,22..23} (4 alike) : BusSelector  OutputSignals=Enable_Wheels
  Bus Selector{11,28..30} (4 alike) : BusSelector  OutputSignals=Steering_Abs_Cmd
  Bus Selector{112..115} (4 alike) : BusSelector  OutputSignals=Swerve_Drive_Integral_Enable
  Bus Selector{2,7,12,14,16,18,20..21,25,50,55,74,79,94,116,121} (16 alike) : BusSelector  OutputSignals=Disabled,Autonomous,Teleop,Test
  Bus Selector{117..120} (4 alike) : BusSelector  OutputSignals=Desired_Pipeline
  Bus Selector{13,31..33} (4 alike) : BusSelector  OutputSignals=Steering_Rel_Cmd
  Bus Selector{15,34..36} (4 alike) : BusSelector  OutputSignals=Translation_Angle
  Bus Selector{17,37..39} (4 alike) : BusSelector  OutputSignals=Translation_Speed
  Bus Selector{19,43..45} (4 alike) : BusSelector  OutputSignals=Is_Absolute_Translation
  Bus Selector{24,26..27,46} (4 alike) : BusSelector  OutputSignals=Is_Absolute_Steering
  Bus Selector{6,8,40..41} (4 alike) : BusSelector  OutputSignals=Spline_Ref_Poses
  Bus Selector{42,48..49,51} (4 alike) : BusSelector  OutputSignals=Spline_Num_Poses
  Bus Selector47 : BusSelector  OutputSignals=PreProcessing
  Bus Selector{52..54,56} (4 alike) : BusSelector  OutputSignals=Test_Mode
  Bus Selector{72..73,75..76} (4 alike) : BusSelector  OutputSignals=Reset_Wheel_Offsets
  Bus Selector{77..78,80..81} (4 alike) : BusSelector  OutputSignals=Disable_Wheels
  Bus Selector{92..93,95..96} (4 alike) : BusSelector  OutputSignals=Swerve_Motors_Disabled
  Merge{1..10,14..16,19,23..24} (16 alike) : Merge  Inputs=4
  Bus_Out : Outport
  wires:
  Bus Selector47/1 -> Bus Creator/17  "<PreProcessing>"
  Merge24/1 -> Bus Creator/16  "Desired_Pipeline"
  Merge23/1 -> Bus Creator/15  "Swerve_Drive_Integral_Enable"
  Bus Selector119/1 -> Merge24/3  "<Desired_Pipeline>"
  Bus Selector118/1 -> Merge24/4  "<Desired_Pipeline>"
  Bus Selector117/1 -> Merge24/2  "<Desired_Pipeline>"
  Bus Selector120/1 -> Merge24/1  "<Desired_Pipeline>"
  Bus Selector121/2 -> Bus Selector117/1  "<Autonomous>"
  Bus Selector121/1 -> Bus Selector120/1  "<Disabled>"
  Bus Selector121/3 -> Bus Selector119/1  "<Teleop>"
  Bus Selector121/4 -> Bus Selector118/1  "<Test>"
  Bus Selector112/1 -> Merge23/2  "<Swerve_Drive_Integral_Enable>"
  Bus Selector116/4 -> Bus Selector114/1  "<Test>"
  Bus Selector113/1 -> Merge23/3  "<Swerve_Drive_Integral_Enable>"
  Bus Selector116/1 -> Bus Selector115/1  "<Disabled>"
  Bus Selector116/3 -> Bus Selector113/1  "<Teleop>"
  Bus Selector116/2 -> Bus Selector112/1  "<Autonomous>"
  Bus Selector114/1 -> Merge23/4  "<Swerve_Drive_Integral_Enable>"
  Bus Selector115/1 -> Merge23/1  "<Swerve_Drive_Integral_Enable>"
  Merge19/1 -> Bus Creator/14  "Swerve_Motors_Disabled"
  Merge16/1 -> Bus Creator/13  "Disable_Wheels"
  Merge15/1 -> Bus Creator/12  "Reset_Wheel_Offsets"
  Merge14/1 -> Bus Creator/11  "Enable_Wheels"
  Bus Creator/1 -> Bus_Out/1
  Bus Selector21/4 -> Bus Selector9/1  "<Test>"
  Bus Selector9/1 -> Merge14/4  "<Enable_Wheels>"
  Bus Selector21/3 -> Bus Selector23/1  "<Teleop>"
  Bus Selector21/2 -> Bus Selector22/1  "<Autonomous>"
  Bus Selector10/1 -> Merge14/1  "<Enable_Wheels>"
  Bus_In/1 -> Bus Selector12/1, Bus Selector14/1, Bus Selector16/1, Bus Selector18/1, Bus Selector20/1, Bus Selector25/1, Bus Selector21/1, Bus Selector74/1, Bus Selector121/1, Bus Selector47/1, Bus Selector116/1, Bus Selector94/1, Bus Selector79/1, Bus Selector55/1, Bus Selector50/1, Bus Selector7/1, Bus Selector2/1
  Bus Selector22/1 -> Merge14/2  "<Enable_Wheels>"
  Bus Selector21/1 -> Bus Selector10/1  "<Disabled>"
  Bus Selector23/1 -> Merge14/3  "<Enable_Wheels>"
  Bus Selector94/4 -> Bus Selector92/1  "<Test>"
  Bus Selector93/1 -> Merge19/1  "<Swerve_Motors_Disabled>"
  Bus Selector94/2 -> Bus Selector95/1  "<Autonomous>"
  Bus Selector92/1 -> Merge19/4  "<Swerve_Motors_Disabled>"
  Bus Selector94/3 -> Bus Selector96/1  "<Teleop>"
  Bus Selector94/1 -> Bus Selector93/1  "<Disabled>"
  Bus Selector96/1 -> Merge19/3  "<Swerve_Motors_Disabled>"
  Bus Selector95/1 -> Merge19/2  "<Swerve_Motors_Disabled>"
  Bus Selector81/1 -> Merge16/3  "<Disable_Wheels>"
  Bus Selector79/4 -> Bus Selector77/1  "<Test>"
  Bus Selector79/1 -> Bus Selector78/1  "<Disabled>"
  Bus Selector79/3 -> Bus Selector81/1  "<Teleop>"
  Bus Selector79/2 -> Bus Selector80/1  "<Autonomous>"
  Bus Selector77/1 -> Merge16/4  "<Disable_Wheels>"
  Bus Selector78/1 -> Merge16/1  "<Disable_Wheels>"
  Bus Selector80/1 -> Merge16/2  "<Disable_Wheels>"
  Bus Selector74/4 -> Bus Selector72/1  "<Test>"
  Bus Selector74/2 -> Bus Selector75/1  "<Autonomous>"
  Bus Selector74/1 -> Bus Selector73/1  "<Disabled>"
  Bus Selector75/1 -> Merge15/2  "<Reset_Wheel_Offsets>"
  Bus Selector76/1 -> Merge15/3  "<Reset_Wheel_Offsets>"
  Bus Selector74/3 -> Bus Selector76/1  "<Teleop>"
  Bus Selector72/1 -> Merge15/4  "<Reset_Wheel_Offsets>"
  Bus Selector73/1 -> Merge15/1  "<Reset_Wheel_Offsets>"
  Merge10/1 -> Bus Creator/10  "Test_Mode"
  Bus Selector55/2 -> Bus Selector56/1  "<Autonomous>"
  Bus Selector53/1 -> Merge10/4  "<Test_Mode>"
  Bus Selector54/1 -> Merge10/1  "<Test_Mode>"
  Bus Selector55/1 -> Bus Selector54/1  "<Disabled>"
  Bus Selector55/4 -> Bus Selector53/1  "<Test>"
  Bus Selector56/1 -> Merge10/2  "<Test_Mode>"
  Bus Selector52/1 -> Merge10/3  "<Test_Mode>"
  Bus Selector55/3 -> Bus Selector52/1  "<Teleop>"
  Merge9/1 -> Bus Creator/9  "Spline_Num_Poses"
  Bus Selector48/1 -> Merge9/4  "<Spline_Num_Poses>"
  Bus Selector50/1 -> Bus Selector49/1  "<Disabled>"
  Bus Selector42/1 -> Merge9/3  "<Spline_Num_Poses>"
  Bus Selector49/1 -> Merge9/1  "<Spline_Num_Poses>"
  Bus Selector51/1 -> Merge9/2  "<Spline_Num_Poses>"
  Bus Selector50/4 -> Bus Selector48/1  "<Test>"
  Bus Selector50/3 -> Bus Selector42/1  "<Teleop>"
  Bus Selector50/2 -> Bus Selector51/1  "<Autonomous>"
  Merge8/1 -> Bus Creator/8  "Spline_Ref_Poses"
  Bus Selector7/2 -> Bus Selector8/1  "<Autonomous>"
  Bus Selector7/3 -> Bus Selector40/1  "<Teleop>"
  Bus Selector7/4 -> Bus Selector41/1  "<Test>"
  Bus Selector8/1 -> Merge8/2  "<Spline_Ref_Poses>"
  Bus Selector6/1 -> Merge8/1  "<Spline_Ref_Poses>"
  Bus Selector40/1 -> Merge8/3  "<Spline_Ref_Poses>"
  Bus Selector7/1 -> Bus Selector6/1  "<Disabled>"
  Bus Selector41/1 -> Merge8/4  "<Spline_Ref_Poses>"
  Merge7/1 -> Bus Creator/7  "Spline_Enable"
  Bus Selector5/1 -> Merge7/4  "<Spline_Enable>"
  Bus Selector2/1 -> Bus Selector1/1  "<Disabled>"
  Bus Selector4/1 -> Merge7/3  "<Spline_Enable>"
  Bus Selector1/1 -> Merge7/1  "<Spline_Enable>"
  Bus Selector3/1 -> Merge7/2  "<Spline_Enable>"
  Bus Selector2/4 -> Bus Selector5/1  "<Test>"
  Bus Selector2/3 -> Bus Selector4/1  "<Teleop>"
  Bus Selector2/2 -> Bus Selector3/1  "<Autonomous>"
  Bus Selector29/1 -> Merge1/3  "<Steering_Abs_Cmd>"
  Bus Selector25/2 -> Bus Selector26/1  "<Autonomous>"
  Bus Selector25/3 -> Bus Selector27/1  "<Teleop>"
  Bus Selector14/3 -> Bus Selector32/1  "<Teleop>"
  Bus Selector16/3 -> Bus Selector35/1  "<Teleop>"
  Bus Selector16/4 -> Bus Selector36/1  "<Test>"
  Bus Selector20/1 -> Bus Selector19/1  "<Disabled>"
  Merge1/1 -> Bus Creator/1  "Steering_Abs_Cmd"
  Bus Selector34/1 -> Merge3/2  "<Translation_Angle>"
  Bus Selector17/1 -> Merge4/1  "<Translation_Speed>"
  Bus Selector15/1 -> Merge3/1  "<Translation_Angle>"
  Bus Selector20/2 -> Bus Selector43/1  "<Autonomous>"
  Bus Selector14/1 -> Bus Selector13/1  "<Disabled>"
  Bus Selector20/4 -> Bus Selector45/1  "<Test>"
  Merge5/1 -> Bus Creator/5  "Is_Absolute_Translation"
  Bus Selector36/1 -> Merge3/4  "<Translation_Angle>"
  Bus Selector12/1 -> Bus Selector11/1  "<Disabled>"
  Bus Selector16/2 -> Bus Selector34/1  "<Autonomous>"
  Bus Selector37/1 -> Merge4/2  "<Translation_Speed>"
  Bus Selector25/4 -> Bus Selector46/1  "<Test>"
  Bus Selector18/3 -> Bus Selector38/1  "<Teleop>"
  Bus Selector20/3 -> Bus Selector44/1  "<Teleop>"
  Bus Selector39/1 -> Merge4/4  "<Translation_Speed>"
  Bus Selector16/1 -> Bus Selector15/1  "<Disabled>"
  Bus Selector13/1 -> Merge2/1  "<Steering_Rel_Cmd>"
  Bus Selector30/1 -> Merge1/4  "<Steering_Abs_Cmd>"
  Bus Selector26/1 -> Merge6/2  "<Is_Absolute_Steering>"
  Merge6/1 -> Bus Creator/6  "Is_Absolute_Steering"
  Bus Selector18/1 -> Bus Selector17/1  "<Disabled>"
  Bus Selector45/1 -> Merge5/4  "<Is_Absolute_Translation>"
  Bus Selector12/3 -> Bus Selector29/1  "<Teleop>"
  Bus Selector18/2 -> Bus Selector37/1  "<Autonomous>"
  Bus Selector43/1 -> Merge5/2  "<Is_Absolute_Translation>"
  Bus Selector19/1 -> Merge5/1  "<Is_Absolute_Translation>"
  Bus Selector35/1 -> Merge3/3  "<Translation_Angle>"
  Merge3/1 -> Bus Creator/3  "Translation_Angle"
  Bus Selector28/1 -> Merge1/2  "<Steering_Abs_Cmd>"
  Bus Selector14/2 -> Bus Selector31/1  "<Autonomous>"
  Bus Selector32/1 -> Merge2/3  "<Steering_Rel_Cmd>"
  Merge4/1 -> Bus Creator/4  "Translation_Speed"
  Bus Selector12/2 -> Bus Selector28/1  "<Autonomous>"
  Bus Selector14/4 -> Bus Selector33/1  "<Test>"
  Bus Selector44/1 -> Merge5/3  "<Is_Absolute_Translation>"
  Bus Selector24/1 -> Merge6/1  "<Is_Absolute_Steering>"
  Bus Selector11/1 -> Merge1/1  "<Steering_Abs_Cmd>"
  Bus Selector31/1 -> Merge2/2  "<Steering_Rel_Cmd>"
  Bus Selector27/1 -> Merge6/3  "<Is_Absolute_Steering>"
  Bus Selector25/1 -> Bus Selector24/1  "<Disabled>"
  Bus Selector18/4 -> Bus Selector39/1  "<Test>"
  Bus Selector46/1 -> Merge6/4  "<Is_Absolute_Steering>"
  Bus Selector38/1 -> Merge4/3  "<Translation_Speed>"
  Bus Selector33/1 -> Merge2/4  "<Steering_Rel_Cmd>"
  Bus Selector12/4 -> Bus Selector30/1  "<Test>"
  Merge2/1 -> Bus Creator/2  "Steering_Rel_Cmd"

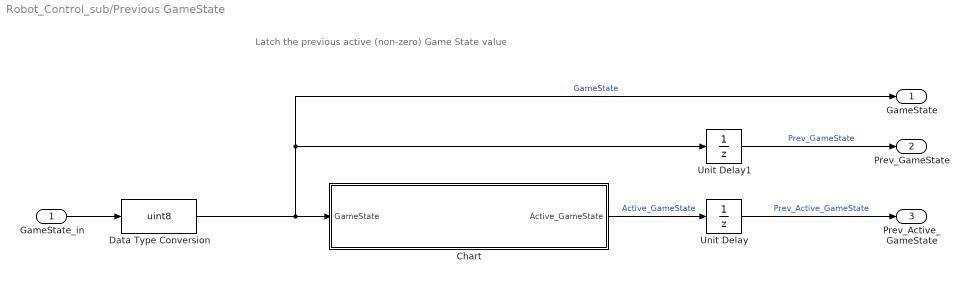
== system Robot_Control_sub/Previous GameState ==
  note: Latch the previous active (non-zero) Game State value
  GameState_in : Inport
  Chart : Stateflow chart  TreatAsAtomicUnit=on
  Data Type Conversion : DataTypeConversion  OutDataTypeStr=uint8  SaturateOnIntegerOverflow=off  RndMeth=Floor
  Unit Delay : UnitDelay  SampleTime=-1  HasFrameUpgradeWarning=on
  Unit Delay1 : UnitDelay  SampleTime=-1  HasFrameUpgradeWarning=on
  GameState : Outport
  Prev_GameState : Outport  Port=2
  Prev_Active_GameState : Outport  Port=3
  wires:
  Unit Delay1/1 -> Prev_GameState/1  "Prev_GameState"
  Chart/1(Active_GameState) -> Unit Delay/1  "Active_GameState"
  Data Type Conversion/1 -> Chart/1(GameState), GameState/1, Unit Delay1/1  "GameState"
  Unit Delay/1 -> Prev_Active_GameState/1  "Prev_Active_GameState"
  GameState_in/1 -> Data Type Conversion/1

== stateflow chart Robot_Control_sub/Previous GameState/Chart ==
  state Disabled
  state Not_Disabled
    en: Active_GameState = GameState;
    du: Active_GameState = GameState;
  (default) -> Disabled : {Active_GameState = 0}
  Disabled -> Not_Disabled : [GameState ~= 0]
  Not_Disabled -> Disabled : [GameState == 0]
  data: GameState input; Active_GameState output
